simulink model "Planta_15_9_24"  (R2021a)
settings: Solver=VariableStepAuto  StartTime=0.0  StopTime=350  FixedStep=0.002  MaxStep=1e-3  RelTol=1e-4
model workspace (MAT data in the model file):
  VelMin = 0.5
  vMax = -0.3
values from neighbouring files (symbols this model uses):
  ax_max = 0.8    [valoresPlanta_29_9_24.m]    (also in valoresPlanta_v4.m)
  ay_max = 0.75    [valoresPlanta_29_9_24.m]    (also in valoresPlanta_v4.m)
  bcy = 1e7    (= 10000000)    [Valores_1.m]    (also in valoresPlanta.m; valoresPlanta_29_9_24.m; valoresPlanta_V3.m; valoresPlanta_v4.m)
  bh_eq = bhm*ih^2+bhd    (= 8720)    [Valores.m]    (also in Valores_1.m; valoresPlanta.m; valoresPlanta_29_9_24.m; valoresPlanta_V3.m)
  bhb = 1e8    (= 100000000)    [Valores.m]    (also in Valores_1.m; valoresPlanta.m; valoresPlanta_29_9_24.m; valoresPlanta_V3.m)
  bhEb = 2.2e9    (= 2200000000)    [Valores.m]    (also in Valores_1.m; valoresPlanta.m; valoresPlanta_29_9_24.m; valoresPlanta_V3.m)
  bt = 90.0    (= 90)    [Valores.m]    (also in Valores_1.m; valoresPlanta.m; valoresPlanta_29_9_24.m; valoresPlanta_V3.m)
  bt_eq = btd+(btm*(it^2))    (= 5401.8)    [valoresPlanta.m]    (also in valoresPlanta_29_9_24.m; valoresPlanta_V3.m; valoresPlanta_v4.m)
  btb = 5e6    (= 5000000)    [Valores.m]    (also in Valores_1.m; valoresPlanta.m; valoresPlanta_29_9_24.m; valoresPlanta_V3.m)
  btw = 3.0e3    (= 3000)    [Valores.m]    (also in Valores_1.m; valoresPlanta.m; valoresPlanta_29_9_24.m; valoresPlanta_V3.m)
  bwu = 150    [Valores.m]    (also in Valores_1.m; valoresPlanta.m; valoresPlanta_29_9_24.m; valoresPlanta_V3.m)
  estado_cont = [x_positions; hy_cont]    [perfilObsaculos.m]    (also in valoresPlanta_29_9_24.m = [x_positions; [hy_muelle hy_cont]]; valoresPlanta_v4.m = [x_positions; [hy_muelle hy_cont]])
  g = 9.80665    [Valores.m]    (also in Valores_1.m; valoresPlanta.m; valoresPlanta_29_9_24.m; valoresPlanta_V3.m)
  Hc = 0    [Valores.m]    (also in Valores_1.m = 2.5; valoresPlanta.m = 2.5; valoresPlanta_29_9_24.m = 2.5; valoresPlanta_V3.m = 2.5)
  hx_cont = 2.5    [perfilObsaculos.m]    (also in puntosTrayectoria.m; valoresPlanta_29_9_24.m; valoresPlanta_v4.m)
  ih = 22    [Valores.m]    (also in Valores_1.m; valoresPlanta.m; valoresPlanta_29_9_24.m; valoresPlanta_V3.m)
  it = 30    [Valores.m]    (also in Valores_1.m; valoresPlanta.m; valoresPlanta_29_9_24.m; valoresPlanta_V3.m)
  Jh_eq = Jhm_hb*ih^2+Jhd_hEb    (= 18320)    [Valores.m]    (also in Valores_1.m; valoresPlanta.m; valoresPlanta_29_9_24.m; valoresPlanta_V3.m)
  Jt_eq = Jtd+(Jtm_tb*(it^2))    (= 7500)    [valoresPlanta.m]    (also in valoresPlanta_29_9_24.m; valoresPlanta_V3.m; valoresPlanta_v4.m)
  kcy = 1.8e9    (= 1800000000)    [Valores_1.m]    (also in valoresPlanta.m; valoresPlanta_29_9_24.m; valoresPlanta_V3.m; valoresPlanta_v4.m)
  KDh = Jeq2 * w_posh^3    (= -12245.4404091)    [Valores.m]    (also in Valores_1.m = Jeq2 * w_posh; valoresPlanta.m = Jeq2 * w_posh; valoresPlanta_29_9_24.m = Jh_eq * n * w_posh; valoresPlanta_V3.m = Jeq2 * w_posh)
  KDt = Meq2 * w_post^3    (= -4728.86946035)    [Valores.m]    (also in Valores_1.m = Meq2 * w_post; valoresPlanta.m = Meq2 * w_post; valoresPlanta_29_9_24.m = 10127; valoresPlanta_V3.m = Meq2 * w_post)
  KIh = Jeq2 * w_posh^2    (= 2572.66592082)    [Valores.m]    (also in Valores_1.m = Jeq2 * w_posh^3; valoresPlanta.m = Jeq2 * w_posh^3; valoresPlanta_29_9_24.m = Jh_eq * w_posh^3; valoresPlanta_V3.m = Jeq2 * w_posh^3)
  KIt = Meq2 * w_post^2    (= 1307.690244)    [Valores.m]    (also in Valores_1.m = Meq2 * w_post^3; valoresPlanta.m = Meq2 * w_post^3; valoresPlanta_29_9_24.m = 6809.6; valoresPlanta_V3.m = Meq2 * w_post^3)
  KPh = Jeq2 * w_posh    (= -540.495867769)    [Valores.m]    (also in Valores_1.m = Jeq2 * w_posh^2; valoresPlanta.m = Jeq2 * w_posh^2; valoresPlanta_29_9_24.m = Jh_eq * n * w_posh^2; valoresPlanta_V3.m = Jeq2 * w_posh^2)
  KPt = Meq2 * w_post    (= -361.62)    [Valores.m]    (also in Valores_1.m = Meq2 * w_post^2; valoresPlanta.m = Meq2 * w_post^2; valoresPlanta_29_9_24.m = 14123; valoresPlanta_V3.m = Meq2 * w_post^2)
  Ktw = 4.8e5    (= 480000)    [Valores.m]    (also in Valores_1.m; valoresPlanta.m; valoresPlanta_29_9_24.m; valoresPlanta_V3.m)
  kwu = 2.36e8    (= 236000000)    [Valores.m]    (also in Valores_1.m; valoresPlanta.m; valoresPlanta_29_9_24.m; valoresPlanta_V3.m)
  Mc_max = 5e4    (= 50000)    [Valores.m]    (also in Valores_1.m; valoresPlanta.m; valoresPlanta_29_9_24.m; valoresPlanta_V3.m)
  Mc_min = 2e3    (= 2000)    [Valores.m]    (also in Valores_1.m; valoresPlanta.m; valoresPlanta_29_9_24.m; valoresPlanta_V3.m)
  Ms = 1.5e4    (= 15000)    [Valores.m]    (also in Valores_1.m; valoresPlanta.m; valoresPlanta_29_9_24.m; valoresPlanta_V3.m)
  Mt = 30000    [Valores.m]    (also in Valores_1.m; valoresPlanta.m; valoresPlanta_29_9_24.m; valoresPlanta_V3.m)
  pos = [p0; p1; p2; p3; p4; p5]    [calcularTrayectoria2_prueba.m]    (also in perfilObsaculos.m = puntosTrayectoria(4, 1.5, 20, [-20,0], estado_cont, hy_cont,; puntosTrayectoria.m; valoresPlanta_29_9_24.m = calcularTrayectoria2_prueba(vx_max, vhmax, ax_max, Hc, hx_co; valoresPlanta_v4.m = calcularTrayectoria2_prueba(vx_max, vhmax, ax_max, Hc, hx_co)
  rhd = 0.75    [Valores.m]    (also in Valores_1.m; valoresPlanta.m; valoresPlanta_29_9_24.m; valoresPlanta_V3.m)
  rtd = 0.5    [Valores.m]    (also in Valores_1.m; valoresPlanta.m; valoresPlanta_29_9_24.m; valoresPlanta_V3.m)
  tau_hm = 1e-3    (= 0.001)    [valoresPlanta.m]    (also in valoresPlanta_29_9_24.m; valoresPlanta_V3.m; valoresPlanta_v4.m)
  tau_tm = 1e-3    (= 0.001)    [Valores.m]    (also in Valores_1.m; valoresPlanta.m; valoresPlanta_29_9_24.m; valoresPlanta_V3.m)
  Thb_Max = 5e4    (= 50000)    [Valores.m]    (also in Valores_1.m; valoresPlanta.m; valoresPlanta_29_9_24.m; valoresPlanta_V3.m)
  ThEb_Max = 1.1e6    (= 1100000)    [Valores.m]    (also in Valores_1.m; valoresPlanta.m; valoresPlanta_29_9_24.m; valoresPlanta_V3.m)
  Thm_Max = 2e4    (= 20000)    [Valores.m]    (also in Valores_1.m; valoresPlanta.m; valoresPlanta_29_9_24.m; valoresPlanta_V3.m)
  Ttb_Max = 5e3    (= 5000)    [Valores.m]    (also in Valores_1.m; valoresPlanta.m; valoresPlanta_29_9_24.m; valoresPlanta_V3.m)
  Ttm_Max = 3e3    (= 3000)    [Valores.m]    (also in Valores_1.m; valoresPlanta.m; valoresPlanta_29_9_24.m = 4000; valoresPlanta_V3.m)
  vhmax = 3    [valoresPlanta_29_9_24.m]    (also in valoresPlanta_V3.m; valoresPlanta_v4.m)
  vx_max = 4    [valoresPlanta_29_9_24.m]    (also in valoresPlanta_v4.m)
  whmMax = P/Thm_Max    (= 47.8075)    [Valores_1.m]    (also in valoresPlanta.m; valoresPlanta_29_9_24.m = 176; valoresPlanta_V3.m; valoresPlanta_v4.m = 176)
  whmMin = 0.02    [valoresPlanta_29_9_24.m]    (also in valoresPlanta_v4.m = 0.2)
  wtmMax = (4/rtd)*it    (= 240)    [Valores_1.m]    (also in valoresPlanta.m; valoresPlanta_29_9_24.m; valoresPlanta_V3.m; valoresPlanta_v4.m)
  wtmMin = 0.02    [valoresPlanta_29_9_24.m]    (also in valoresPlanta_v4.m = 0.2)
  x_0 = -20    [valoresPlanta_29_9_24.m]    (also in valoresPlanta_v4.m)
  x_0_tamb = x_0/rtd    (= -40)    [valoresPlanta_29_9_24.m]    (also in valoresPlanta_v4.m)
  xLimMax = 49    [valoresPlanta_29_9_24.m]    (also in valoresPlanta_v4.m)
  xLimMaxSeguridad = 50    [valoresPlanta_29_9_24.m]    (also in valoresPlanta_v4.m)
  xLimMin = -29    [valoresPlanta_29_9_24.m]    (also in valoresPlanta_v4.m)
  xLimMinSeguridad = -30    [valoresPlanta_29_9_24.m]    (also in valoresPlanta_v4.m)
  y_0 = 2.5    [valoresPlanta_29_9_24.m]    (also in valoresPlanta_v4.m)
  y_0_izaje = 3*(2/rhd)    (= 8)    [valoresPlanta_29_9_24.m]    (also in valoresPlanta_v4.m)
  yLimMax = 44    [valoresPlanta_29_9_24.m]    (also in valoresPlanta_v4.m)
  yLimMaxSeguridad = 45    [valoresPlanta_29_9_24.m]    (also in valoresPlanta_v4.m)
  yLimMin = -19    [valoresPlanta_29_9_24.m]    (also in valoresPlanta_v4.m)
  yLimMinSeguridad = -20    [valoresPlanta_29_9_24.m]    (also in valoresPlanta_v4.m)
  Yt0 = 45    [Valores.m]    (also in Valores_1.m; valoresPlanta.m; valoresPlanta_29_9_24.m; valoresPlanta_V3.m)
undefined symbols (not defined in the file or in its folder): DiscIntNeverNeededParam
libraries: simulink x4, vrlib x1, simulink_extras x1, aerolibanimutils x1
(part 1 of 3)
settings Model: Creator=Matias  LastModifiedBy=agustin

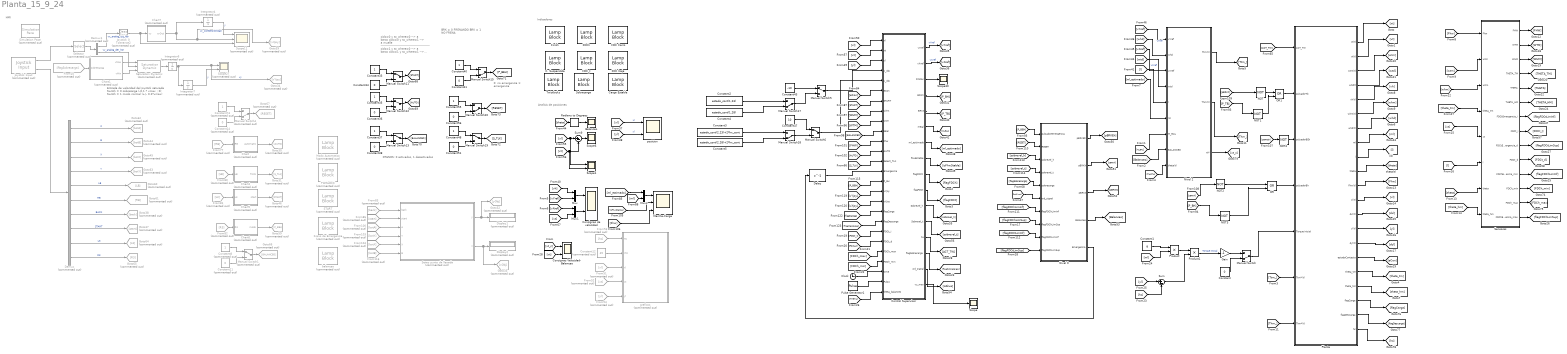
== system Planta_15_9_24 ==
  note: Entrada de velocidad del joystick saturada
      | Switch = 0 sobrecarga (-0.1 * vmax ; 0)
      | Switch = 1 modo normal (+/- 0.2*vmax)
  note: Indicadores
  note: Analisis de posiciones
  note: HMI
  note: 0: no emergencia
      | 1: emergencia
  note: ciclo=0 y to_where=0 --> a barco
      | ciclo=0 y to_where=1 --> a muelle
      | -------------------------------------------------
      | ciclo=1 y to_where=0 --> a barco
      | ciclo=1 y to_where=1 --> a barco 2
      | ciclo=1 y to_where=2 --> a muelle
  note: FRENOS: 0 activados, 1 desactivados
  note: BRK = 0 FRENANDO
      | BRK = 1 NO FRENA
  Balanceo : Scope
  C. Suspendida : LampBlock
  Carga Estable : LampBlock
  Chart : Stateflow chart  Commented=on  TreatAsAtomicUnit=on
  Chart1 : Stateflow chart  Commented=on  TreatAsAtomicUnit=on
  Chart4 : Stateflow chart  Commented=on  TreatAsAtomicUnit=on
  Chart5 : Stateflow chart  Commented=on  TreatAsAtomicUnit=on
  Chart6 : Stateflow chart  Commented=on  TreatAsAtomicUnit=on
  Chart7 : Stateflow chart  Commented=on  TreatAsAtomicUnit=on
  Clock : Clock
  Consignas Velocidad-Balanceo : Scope  NumInputPorts=2
  Consignas de velocidad : Scope  NumInputPorts=2
  Constant{,34,36,38,41,51,56} (7 alike) : Constant  Value=0
  Constant1 : Constant  Value=g
  Constant11 : Constant  Commented=on  Value=0
  Constant12 : Constant  Commented=on  Value=45
  Constant13 : Constant  Commented=on
  Constant14 : Constant  Commented=on  Value=0
  Constant2 : Constant  Value=estado_cont(1,23)
  Constant3 : Constant  Value=estado_cont(2,23)+2*hx_cont
  Constant{33,35,37,40,48,55} (6 alike) : Constant
  Constant4 : Constant  Value=estado_cont(1,28)
  Constant43 : Constant  Value=-10
  Constant47 : Constant  Value=10
  Constant5 : Constant  Value=estado_cont(2,28)+2*hx_cont
  Constant8 : Constant  Commented=on
  Control Supervisor : Subsystem  TreatAsAtomicUnit=on  SystemSampleTime=0.02
  Delay : Delay  DelayLength=1  InputProcessing=Columns as channels (frame based)
  Demux : Demux  Commented=on  Outputs=10
  Demux1 : Demux  Commented=on  Outputs=2
  Display1 : Display  Commented=on
  Display2 : Display  Commented=on
  FDC Carro : LampBlock
  FDC Izaje : LampBlock
  FDC_t : LampBlock
  FDCh : LampBlock
  Finish : LampBlock
  Freno de Emergencia : LampBlock  Commented=on  LabelPosition=Hide
  From10 : From  Commented=on  GotoTag=flagSobrecarga
  From100 : From  Commented=on  GotoTag=botA
  From103 : From  Commented=on  GotoTag=botY
  From104 : From  Commented=on  GotoTag=botX
  From116 : From  Commented=on  GotoTag=botB
  From51 : From  Commented=on  GotoTag=xl
  From52 : From  Commented=on  GotoTag=xt
  From53 : From  Commented=on  GotoTag=hc
  From54 : From  Commented=on  GotoTag=yl
  From77 : From  Commented=on  GotoTag=RB
  From80 : From  Commented=on  GotoTag=LB
  From81 : From  Commented=on  GotoTag=L3
  From82 : From  Commented=on  GotoTag=R3
  From83 : From  Commented=on  GotoTag=back
  From86 : From  Commented=on  GotoTag=start
  Gain : Gain  Gain=-1
  Goto30 : Goto  Commented=on  GotoTag=AUTO
  Goto31 : Goto  Commented=on  GotoTag=S_TLK
  Goto32 : Goto  Commented=on  GotoTag=yObj
  Goto33 : Goto  Commented=on  GotoTag=xObj
  Goto34 : Goto  Commented=on  GotoTag=vYjoy
  Goto37 : Goto  Commented=on  GotoTag=start
  Goto38 : Goto  Commented=on  GotoTag=back
  Goto39 : Goto  Commented=on  GotoTag=vXjoy
  Goto44 : Goto  Commented=on  GotoTag=botB
  Goto45 : Goto  Commented=on  GotoTag=botX
  Goto46 : Goto  Commented=on  GotoTag=START
  Goto59 : Goto  Commented=on  GotoTag=P_BEH
  Goto60 : Goto  Commented=on  GotoTag=LB
  Goto61 : Goto  Commented=on  GotoTag=RB
  Goto62 : Goto  Commented=on  GotoTag=botA
  Goto63 : Goto  Commented=on  GotoTag=botY
  Goto64 : Goto  Commented=on  GotoTag=L3
  Goto65 : Goto  Commented=on  GotoTag=R3
  Goto66 : Goto  Commented=on  GotoTag=BALANCEO
  Goto67 : Goto  Commented=on  GotoTag=RESET
  Integrator4 : Integrator  Commented=on
  Integrator6 : Integrator  Commented=on  InitialCondition=[0]  LimitOutput=on  UpperSaturationLimit=[3.5]  LowerSaturationLimit=[-3.5]
  Integrator7 : Integrator  Commented=on
  Joystick 0 Tolerance2 : DeadZone  Commented=on  LowerValue=-0.2  UpperValue=0.2  SaturateOnIntegerOverflow=on
  Joystick Input : vrlib/Joystick Input  Commented=on  joyid=1  adjustports=on  forcefeed=off
  Manual Switch{,15,17..18,20} (5 alike) : ManualSwitch  CurrentSetting=0
  Manual Switch1 : ManualSwitch  Commented=on
  Manual Switch{5..6,11..13,19} (6 alike) : ManualSwitch
  Manual Switch4 : ManualSwitch  Commented=on  CurrentSetting=0
  Marcha-Carga : Scope  NumInputPorts=3
  Modo Automatico : LampBlock  Commented=on  LabelPosition=Hide
  Mux : Mux  Inputs=2
  Mux1 : Mux  Inputs=2
  Mux2 : Mux  Inputs=2
  NOT{,1..4} (5 alike) : Logic  Operator=NOT  IconShape=distinctive  AllPortsSameDT=off  OutDataTypeStr=boolean
  Nivel 0 : Stateflow chart  TreatAsAtomicUnit=on  SystemSampleTime=0.02
  Nivel 2 : Subsystem  SystemSampleTime=0.005
  OR : Logic  Operator=OR  IconShape=distinctive  AllPortsSameDT=off  OutDataTypeStr=fixdt(0,1)
  OR1 : Logic  Operator=OR  IconShape=distinctive  AllPortsSameDT=off  OutDataTypeStr=fixdt(0,1)
  Planta : Subsystem
  Product : Product
  Product1 : Product
  Pulse Generator1 : DiscretePulseGenerator  PulseType=Time based  Period=1  PulseWidth=50
  Radians to Degrees : simulink_extras/Transformations/Radians to Degrees
  START : LampBlock  Commented=on  LabelPosition=Hide
  Saturation Dynamic : simulink/Discontinuities/Saturation Dynamic  Commented=on  OutMin=[]  OutMax=[]  OutDataTypeStr=Inherit: Same as second input  OutDataType=fixdt(1, 16)  OutScaling=2^-10  DoSatur=off
  Scope : Scope
  Scope1 : Scope  NumInputPorts=2
  Scope11 : Scope  Commented=on  NumInputPorts=3
  Scope27 : Scope  Commented=on  NumInputPorts=2
  Scope30 : Scope
  Scope6 : Scope
  Selector : Selector  Commented=on  InputPortWidth=5  IndexOptions=Index vector (dialog)  Indices=[1 4]  OutputSizes=1
  Sensores : Subsystem
  Seteo punto de llegada : Stateflow chart  Commented=on  TreatAsAtomicUnit=on
  Simulation Pace : aerolibanimutils/Simulation Pace  Commented=on  SimulationPace=1  SleepMode=Auto  OutputPaceError=off  SampleTime=1/50
  Sobrecarga : LampBlock
  Sum : Sum  Inputs=|+-
  Sum9 : Sum  Inputs=|+-
  TWISLOCK : LampBlock  Commented=on  LabelPosition=Hide
  Twistlocks : LampBlock
  balanceo : LampBlock  Commented=on  LabelPosition=Hide
  graficos : Stateflow chart  Commented=on  TreatAsAtomicUnit=on
  posicion : Scope  NumInputPorts=2
  wires:
  [xl] -> posicion/1  "xl"
  [yl] -> posicion/2  "yl"
  [yl] -> Control Supervisor/3(yl)
  Control Supervisor/2(vXref) -> [vXref]  "vXref"
  Control Supervisor/1(vYref) -> [vYref]  "vYref"
  [xl] -> Control Supervisor/1(xl)
  Constant12/1 -> graficos/2(Yt0)
  From52/1 -> graficos/4(xt)
  From51/1 -> graficos/3(xl)
  From53/1 -> graficos/1(Hc)
  From54/1 -> graficos/5(yl)
  [xl] -> Scope1/1, Sum9/1
  [xt] -> Sum9/2, Scope1/2
  Sum9/1 -> Scope6/1
  Radians to Degrees/1 -> Balanceo/1
  [theta] -> Radians to Degrees/1
  [xt] -> Control Supervisor/2(xt)
  [vh] -> Mux/1
  [vt] -> Mux1/2
  Mux1/1 -> Consignas de velocidad/2
  Mux/1 -> Consignas de velocidad/1
  [START] -> Control Supervisor/7(START)
  Control Supervisor/3(FINISH) -> Scope30/1
  [P_TB] -> NOT1/1
  [P_BH] -> NOT3/1
  [eCon] -> Control Supervisor/6(eCon)
  [WTM] -> Control Supervisor/9(wtm)
  [WHM] -> Control Supervisor/8(whm)
  [BALANCEO] -> Control Supervisor/10(bBal)
  Control Supervisor/6(mBal) -> [M_BAL]
  Control Supervisor/5(BRKt) -> [P_TB]
  Control Supervisor/4(BRKh) -> [P_BH]
  [FHW] -> Control Supervisor/11(Fhw)
  [AUTO] -> Control Supervisor/12(AUTO)
  [S_TLK] -> Control Supervisor/13(Select_TLK)
  Control Supervisor/7(ml_estimado) -> [ml_estimado]
  [ml] -> Mux2/2
  [ml_estimado] -> Mux2/1
  Control Supervisor/8(fhwEstable) -> [isFhwStable]
  [isFhwStable] -> Marcha-Carga/2
  [Fhw] -> Marcha-Carga/3
  [P_BEH] -> Nivel 0/1(pulsadorEmergencia)
  Nivel 0/3(pBRKt) -> [pBRKt]
  Nivel 0/2(pBRKh) -> [pBRKh]
  Nivel 0/1(pBRKEh) -> [pBRKEh]
  [pBRKh] -> NOT2/1
  [pBRKt] -> NOT/1
  Nivel 0/4(Balanceo) -> [Balanceo]
  Control Supervisor/9(flagFDCh) -> [flagFDCh]
  Control Supervisor/10(flagFDCt) -> [flagFDCt]
  [RESET] -> Nivel 0/2(RESET)
  Control Supervisor/11(Sobrevel_h) -> [sobrevel_h]
  Control Supervisor/12(Sobrevel_t) -> [sobrevel_t]
  [sobrevel_t] -> Nivel 0/4(sobrevel_t)
  [sobrevel_h] -> Nivel 0/3(sobrevel_h)
  Delay/1 -> Control Supervisor/14(Emergencia)
  [P_BEH] -> Control Supervisor/15(P_EH)
  Nivel 0/5(Emergencia) -> Delay/1
  Control Supervisor/13(tw) -> [ACT_TW]
  [flagSobrecarga] -> Nivel 0/5(sobrecarga)
  From83/1 -> Seteo punto de llegada/1(back)
  From86/1 -> Seteo punto de llegada/2(start)
  Chart7/1(vyOut) -> Goto39/1, Scope11/2, Integrator4/1  "vy_conSensibilidad"
  Seteo punto de llegada/1(y) -> Goto32/1, Display1/1
  Seteo punto de llegada/2(x) -> Goto33/1, Display2/1
  Chart4/1(TWIS) -> Goto31/1
  From100/1 -> Seteo punto de llegada/3(A)
  From104/1 -> Seteo punto de llegada/5(X)
  Demux/9 -> Goto64/1  "L3"
  From103/1 -> Seteo punto de llegada/4(Y)
  Selector/1 -> Demux1/1
  Integrator7/1 -> Scope27/2  "y"
  Integrator4/1 -> Scope11/1  "y"
  Demux1/2 -> Saturation Dynamic/2  "vy_analog_der_hor"
  From80/1 -> Chart4/1(LB)
  Demux1/1 -> Joystick 0 Tolerance2/1  "vx_analog_izq_hor"
  Demux/5 -> Goto60/1  "LB"
  From81/1 -> Chart5/1(L3)
  From82/1 -> Chart6/1(R3)
  Chart5/1(start) -> Goto46/1
  Saturation Dynamic/1 -> Integrator6/1
  Integrator6/1 -> Integrator7/1, Goto34/1, Scope27/1  "vy"
  Demux/10 -> Goto65/1  "R3"
  Chart/1(automatic) -> Goto30/1
  Joystick Input/1 -> Selector/1
  Chart6/1(modo) -> Goto59/1
  From77/1 -> Chart/1(RB)
  Demux/8 -> Goto37/1  "START"
  Demux/3 -> Goto45/1  "X"
  From116/1 -> Seteo punto de llegada/6(B)
  Demux/4 -> Goto63/1  "Y"
  Joystick Input/2 -> Demux/1
  Demux/6 -> Goto61/1  "RB"
  Demux/7 -> Goto38/1  "BACK"
  Demux/1 -> Goto62/1  "A"
  Demux/2 -> Goto44/1  "B"
  Joystick 0 Tolerance2/1 -> Scope11/3, Chart7/1(vy)
  Manual Switch1/1 -> Goto66/1
  Constant8/1 -> Manual Switch1/1
  Constant11/1 -> Manual Switch1/2
  Manual Switch4/1 -> Goto67/1
  Constant14/1 -> Manual Switch4/2
  Constant13/1 -> Manual Switch4/1
  [vYjoy] -> Control Supervisor/16(vYjoy)
  [vXjoy] -> Control Supervisor/17(vXjoy)
  [flagCarga] -> Control Supervisor/18(flagCarga)
  Control Supervisor/14(flagSobrecarga) -> [flagSobrecarga]
  Control Supervisor/15(wd_signal) -> [isAlive]
  [isAlive] -> Nivel 0/6(wd_signal)
  Manual Switch11/1 -> [START]
  Constant56/1 -> Manual Switch20/2
  Constant51/1 -> Manual Switch19/2
  Manual Switch19/1 -> [S_TLK]
  Constant37/1 -> Manual Switch13/1
  Constant48/1 -> Manual Switch19/1
  Constant55/1 -> Manual Switch20/1
  Manual Switch12/1 -> [AUTO]
  Manual Switch13/1 -> [BALANCEO]
  Constant40/1 -> Manual Switch15/1
  Manual Switch20/1 -> [RESET]
  Constant41/1 -> Manual Switch15/2
  Constant36/1 -> Manual Switch12/2
  Constant33/1 -> Manual Switch11/1
  Manual Switch15/1 -> [P_BEH]
  Constant35/1 -> Manual Switch12/1
  Constant34/1 -> Manual Switch11/2
  Constant38/1 -> Manual Switch13/2
  Constant2/1 -> Manual Switch17/1
  Constant3/1 -> Manual Switch18/1
  Constant43/1 -> Manual Switch5/1
  Manual Switch17/1 -> Manual Switch5/2
  Manual Switch5/1 -> Control Supervisor/4(x_obj)
  Manual Switch6/1 -> Control Supervisor/5(y_obj)
  Manual Switch18/1 -> Manual Switch6/2
  Constant47/1 -> Manual Switch6/1
  [flagDescarga] -> Control Supervisor/19(flagDescarga)
  [ACT_TW] -> Planta/1(ACT_TW)
  Planta/1(xt(t)) -> [xt]
  Planta/2(vt(t)) -> [vt]
  Planta/3(wtm(t)) -> [wtm]
  Planta/4(wtd(t)) -> [wtd]
  Planta/5(vh(t)) -> [vh]
  Planta/6(whm(t)) -> [whm]
  Planta/7(whd(t)) -> [whd]
  Planta/8(ml) -> [ml]
  Planta/9(l) -> [l]
  Planta/10(theta) -> [theta]
  Planta/11(Fhw(t)) -> [Fhw]
  Planta/12(xl(t)) -> [xl]
  Planta/13(dxl(t)) -> [dxl]
  Planta/14(yl(t)) -> [yl]
  Planta/15(dyl(t)) -> [dyl]
  [pBRKEh] -> NOT4/1
  OR/1 -> Planta/4(pulsadorBh)
  OR1/1 -> Planta/2(pulsadorTb)
  [vYref] -> Nivel 2/1(vYref)  "vYref"
  [whd] -> Nivel 2/2(whd)
  [vXref] -> Nivel 2/3(vXref)  "vXref"
  [wtd] -> Nivel 2/4(wtd)
  [ml_estimado] -> Nivel 2/6(ml)
  Nivel 2/1(Ttm(t)) -> [Ttm_]
  Nivel 2/2(Thm(t)) -> [Thm_]
  [l] -> Nivel 2/5(l)
  [Balanceo] -> Nivel 2/8(BALANCEO)
  [M_BAL] -> Nivel 2/7(M_BAL)
  [vYref] -> Mux/2
  [vXref] -> Mux1/1
  Planta/16(estadoContacto) -> [eCon]
  [Fhw] -> Sensores/1(Fhw)
  From10/1 -> Chart1/1(sobreCarga)
  Chart1/1(vMax) -> Saturation Dynamic/1
  Chart1/2(vMin) -> Saturation Dynamic/3
  [wtm] -> Sensores/2(wtm)
  [whm] -> Sensores/3(whm)
  [theta] -> Sensores/7(theta)
  Planta/18(theta_hm) -> [theta_hm]
  Planta/17(theta_tm) -> [theta_tm]
  [theta_tm] -> Sensores/4(theta_tm)
  [theta_hm] -> Sensores/8(theta_hm)
  [xt] -> Sensores/5(xt)
  [l] -> Sensores/6(l)
  Sensores/1(FHW) -> [FHW]
  Sensores/2(WTM) -> [WTM]
  Sensores/3(WHM) -> [WHM]
  Sensores/4(THETA_TM) -> [THETA_TM]
  Sensores/5(THETA) -> [THETA]
  Sensores/6(THETA_HM) -> [THETA_HM]
  [flagFDChLimInf] -> Nivel 0/7(flagFDChLimInf)
  [flagFDChLimSup] -> Nivel 0/8(flagFDChLimSup)
  [flagFDCtLimInf] -> Nivel 0/9(flagFDCtLimInf)
  [flagFDCtLimSup] -> Nivel 0/10(flagFDCtLimSup)
  Sensores/11(FDChEmergencia_min) -> [flagFDChLimInf]
  Sensores/9(FDCtEmergencia_d) -> [flagFDCtLimSup]
  Sensores/7(FDCtEmergencia_i) -> [flagFDCtLimInf]
  Sensores/14(FDChEmergencia_max) -> [flagFDChLimSup]
  Sensores/13(FDCh_max) -> [FDCh_max]
  Sensores/12(FDCh_min) -> [FDCh_min]
  Sensores/10(FDCt_d) -> [FDCt_d]
  Sensores/8(FDCt_i) -> [FDCt_i]
  [FDCt_i] -> Control Supervisor/20(FDCt_i)
  [FDCt_d] -> Control Supervisor/21(FDCt_d)
  [FDCh_max] -> Control Supervisor/22(FDCh_max)
  [FDCh_min] -> Control Supervisor/23(FDCh_min)
  Planta/19(flagCarga) -> [flagCarga]
  Planta/20(flagDescarga) -> [flagDescarga]
  Constant1/1 -> Product/1
  [ml] -> Product/2
  Product/1 -> Product1/1
  [yl] -> Sum/1
  [hc] -> Sum/2
  Sum/1 -> Product1/2
  Product1/1 -> Gain/1  "Torque Inicial"
  Planta/21(hc) -> [hc]
  Manual Switch/1 -> Planta/5(Torque Inicial)
  Constant/1 -> Manual Switch/2
  Gain/1 -> Manual Switch/1
  NOT1/1 -> OR1/2
  NOT/1 -> OR1/1
  NOT3/1 -> OR/2
  NOT2/1 -> OR/1
  NOT4/1 -> Planta/3(pulsadorBEh)
  Clock/1 -> Control Supervisor/24(time)
  Pulse Generator1/1 -> Control Supervisor/25(Pulso)
  [Thm_] -> Planta/7(Thm*(t))
  [Ttm_] -> Planta/6(Ttm*(t))
  Control Supervisor/16(vy_max) -> Scope/1
  [THETA] -> Nivel 2/9(theta(t))
  [THETA] -> Control Supervisor/26(theta_balanceo)
  Nivel 2/3(xt*) -> [xt_c]
  [xt_c] -> Consignas Velocidad-Balanceo/1
  [vt] -> Consignas Velocidad-Balanceo/2
  Mux2/1 -> Marcha-Carga/1
  Constant5/1 -> Manual Switch18/2
  Constant4/1 -> Manual Switch17/2

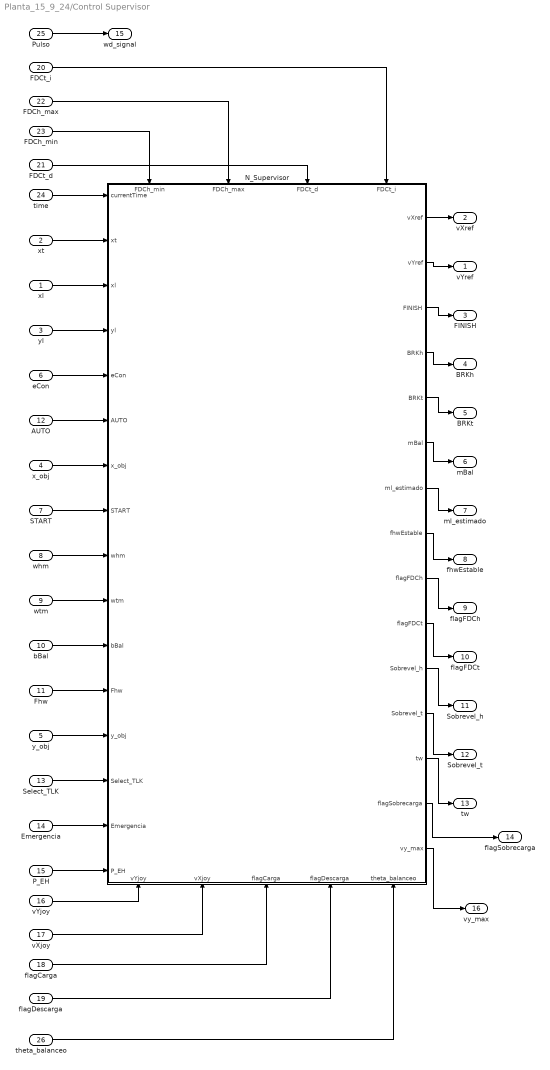
== system Planta_15_9_24/Control Supervisor ==
  xl : Inport
  xt : Inport  Port=2
  yl : Inport  Port=3
  x_obj : Inport  Port=4
  y_obj : Inport  Port=5
  eCon : Inport  Port=6
  START : Inport  Port=7
  whm : Inport  Port=8
  wtm : Inport  Port=9
  bBal : Inport  Port=10
  Fhw : Inport  Port=11
  AUTO : Inport  Port=12
  Select_TLK : Inport  Port=13
  Emergencia : Inport  Port=14
  P_EH : Inport  Port=15
  vYjoy : Inport  Port=16
  vXjoy : Inport  Port=17
  flagCarga : Inport  Port=18
  flagDescarga : Inport  Port=19
  FDCt_i : Inport  Port=20
  FDCt_d : Inport  Port=21
  FDCh_max : Inport  Port=22
  FDCh_min : Inport  Port=23
  time : Inport  Port=24
  Pulso : Inport  Port=25
  theta_balanceo : Inport  Port=26
  N_Supervisor : Stateflow chart  TreatAsAtomicUnit=on
      settings: PortSchema="{\"entries\":[{\"content\":{\"sides\":[{\"content\":{\"connectorIds\":[\"In13\",\"In11\",\"In8\",\"In10\",\"In12\",\"In19\",\"In20\",\"In14\",\"In15\",\"In16\",\"In17\",\"In18\",\"In21\",\"In22\",\"In23\",\"In24\"]},\"type\":\"ConnectorPlacement.EquallySpacedRectSide\",\"uuid\":\"7754e6e1-1487-4c5e-b93c-5b95548dc503\"},{\"content\":{\"connectorIds\":[\"Out1\",\"Out2\",\"Out3\",\"Out4\",\"Out5\",\"Out6\",\"Out7\",\"Out8\",\"Out9\",\"Out10\",\"Out11\",\"Out12\",\"Out13\",\"Out14\",\"Out15\"],\"side\":\"RIGHT\"},\"type\":\"ConnectorPlacement.EquallySpacedRectSide\",\"uuid\":\"e49bdf6e-b30d-4ce2-b56a-406d79434d70\"},{\"content\":{\"connectorIds\":[\"In1\",\"In2\",\"In3\",\"In4\"],\"side\":\"TOP\"},\"type\":\"ConnectorPlacement.EquallySpacedRectSide\",\"uuid\":\"816dde99-88b4-4e51-8e7c-8334ef27840c\"},{\"content\":{\"connectorIds\":[\"In6\",\"In7\",\"In25\",\"In9\",\"In5\"],\"side\":\"BOTTOM\"},\"type\":\"ConnectorPlacement.EquallySpacedRectSide\",\"uuid\":\"e82c3757-072b-4fbd-890b-1ff74979e1d6\"}]},\"type\":\"ConnectorPlacement.EquallySpacedConnector\",\"uuid\":\"e43ca6b0-ace3-4be2-8389-da1b8832a6a4\"}],\"packageUris\":[\"http://schema.mathworks.com/mf0/Connector/R2020b\"],\"version\":\"1.0\"}"
  vYref : Outport
  vXref : Outport  Port=2
  FINISH : Outport  Port=3
  BRKh : Outport  Port=4
  BRKt : Outport  Port=5
  mBal : Outport  Port=6
  ml_estimado : Outport  Port=7
  fhwEstable : Outport  Port=8
  flagFDCh : Outport  Port=9
  flagFDCt : Outport  Port=10
  Sobrevel_h : Outport  Port=11
  Sobrevel_t : Outport  Port=12
  tw : Outport  Port=13
  flagSobrecarga : Outport  Port=14
  wd_signal : Outport  Port=15
  vy_max : Outport  Port=16
  wires:
  N_Supervisor/3(FINISH) -> FINISH/1
  flagCarga/1 -> N_Supervisor/25(flagCarga)
  N_Supervisor/8(fhwEstable) -> fhwEstable/1
  flagDescarga/1 -> N_Supervisor/9(flagDescarga)
  N_Supervisor/4(BRKh) -> BRKh/1
  N_Supervisor/9(flagFDCh) -> flagFDCh/1
  Pulso/1 -> wd_signal/1
  FDCh_max/1 -> N_Supervisor/2(FDCh_max)
  N_Supervisor/6(mBal) -> mBal/1
  N_Supervisor/13(tw) -> tw/1
  FDCt_i/1 -> N_Supervisor/4(FDCt_i)
  time/1 -> N_Supervisor/13(currentTime)
  N_Supervisor/2(vYref) -> vYref/1
  FDCh_min/1 -> N_Supervisor/1(FDCh_min)
  N_Supervisor/1(vXref) -> vXref/1
  Emergencia/1 -> N_Supervisor/23(Emergencia)
  FDCt_d/1 -> N_Supervisor/3(FDCt_d)
  Fhw/1 -> N_Supervisor/18(Fhw)
  P_EH/1 -> N_Supervisor/24(P_EH)
  vXjoy/1 -> N_Supervisor/7(vXjoy)
  vYjoy/1 -> N_Supervisor/6(vYjoy)
  whm/1 -> N_Supervisor/15(whm)
  N_Supervisor/14(flagSobrecarga) -> flagSobrecarga/1
  N_Supervisor/5(BRKt) -> BRKt/1
  N_Supervisor/12(Sobrevel_t) -> Sobrevel_t/1
  eCon/1 -> N_Supervisor/12(eCon)
  N_Supervisor/11(Sobrevel_h) -> Sobrevel_h/1
  xt/1 -> N_Supervisor/11(xt)
  bBal/1 -> N_Supervisor/17(bBal)
  xl/1 -> N_Supervisor/8(xl)
  N_Supervisor/10(flagFDCt) -> flagFDCt/1
  wtm/1 -> N_Supervisor/16(wtm)
  N_Supervisor/7(ml_estimado) -> ml_estimado/1
  AUTO/1 -> N_Supervisor/19(AUTO)
  Select_TLK/1 -> N_Supervisor/22(Select_TLK)
  x_obj/1 -> N_Supervisor/20(x_obj)
  yl/1 -> N_Supervisor/10(yl)
  y_obj/1 -> N_Supervisor/21(y_obj)
  START/1 -> N_Supervisor/14(START)
  N_Supervisor/15(vy_max) -> vy_max/1
  theta_balanceo/1 -> N_Supervisor/5(theta_balanceo)

== system Planta_15_9_24/Nivel 2 ==
  vYref : Inport
  whd : Inport  Port=2
  vXref : Inport  Port=3
  wtd : Inport  Port=4
  l : Inport  Port=5
  ml : Inport  Port=6
  M_BAL : Inport  Port=7
  BALANCEO : Inport  Port=8
  theta(t) : Inport  Port=9
  Subsystem1 : Subsystem  TreatAsAtomicUnit=on  SystemSampleTime=0.005
  Ttm(t) : Outport
  Thm(t) : Outport  Port=2
  xt* : Outport  Port=3
  wires:
  vYref/1 -> Subsystem1/1(vYref)
  M_BAL/1 -> Subsystem1/7(M_BAL)
  whd/1 -> Subsystem1/2(whd)
  BALANCEO/1 -> Subsystem1/8(BALANCEO)
  vXref/1 -> Subsystem1/3(vXref)
  wtd/1 -> Subsystem1/4(wtd)
  l/1 -> Subsystem1/5(l)
  ml/1 -> Subsystem1/6(ml)
  Subsystem1/2(Thm_) -> Thm(t)/1
  Subsystem1/1(Ttm_) -> Ttm(t)/1
  theta(t)/1 -> Subsystem1/9(theta(t))
  Subsystem1/3(xt*) -> xt*/1

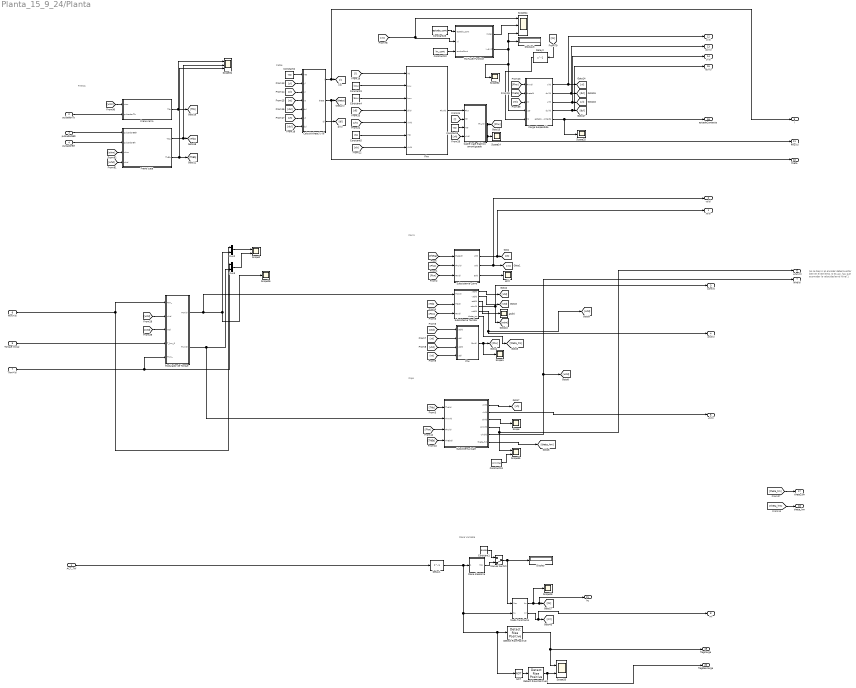
== system Planta_15_9_24/Planta ==
  note: No se bien si el encoder debería estar bien en el eje lento. Si es asi, hay que acomodar la velocidad en el Nivel 1
  note: Masa Variable
  note: Cable
  note: Izaje
  note: Carro
  note: Frenos
  ACT_TW : Inport
  pulsadorTb : Inport  Port=2
  pulsadorBEh : Inport  Port=3
  pulsadorBh : Inport  Port=4
  Torque Inicial : Inport  Port=5
  Ttm*(t) : Inport  Port=6
  Thm*(t) : Inport  Port=7
  Cable izaje elástico amortiguado : Subsystem
  Calculo theta,l y dl : Subsystem
  Carga Suspendida : Subsystem
  Constant1 : Constant  Value=50000
  Constant19 : Constant  Value=whmMax
  Constant2 : Constant  Value=Yt0
  Constant22 : Constant  Value=hx_cont
  Constant23 : Constant  Value=estado_cont
  Constant3 : Constant  Value=kwu
  Constant4 : Constant  Value=bwu
  Constant5 : Constant  Value=Yt0
  Constant6 : Constant  Value=Yt0
  Delay1 : Delay  DelayLength=1  InputProcessing=Columns as channels (frame based)
  Delay2 : Delay  DelayLength=1  InputProcessing=Columns as channels (frame based)
  Detect Rise Positive : simulink/Logic and Bit Operations/Detect Rise Positive  vinit=0  OutDataTypeStr=boolean
  Detect Rise Positive1 : simulink/Logic and Bit Operations/Detect Rise Positive  vinit=0  OutDataTypeStr=boolean
  Display : Display
  Display3 : Display
  Fhw : Subsystem
  Freno Izaje : Subsystem
  Freno carro : Subsystem
  Ftw : Subsystem
  MATLAB Function : MATLAB Function  TreatAsAtomicUnit=on
  Manual Switch : ManualSwitch  CurrentSetting=0
  Masa Aleatoria : Stateflow chart  TreatAsAtomicUnit=on
  Modo Twistlocks : Stateflow chart  TreatAsAtomicUnit=on
  Modulador de Torque : Subsystem
  Mux2 : Mux  Inputs=2
  Mux3 : Mux  Inputs=2
  NOT : Logic  Operator=NOT  IconShape=distinctive  AllPortsSameDT=off  OutDataTypeStr=boolean
  Scope{,1,14,25..26,28,32} (7 alike) : Scope
  Scope2 : Scope  NumInputPorts=2
  Scope24 : Scope  NumInputPorts=3
  Scope31 : Scope  NumInputPorts=3
  Scope33 : Scope  NumInputPorts=2
  Scope35 : Scope  NumInputPorts=2
  Subsistema Carro : Subsystem
  Subsistema Izaje : Subsystem
  Subsistema Tambor : Subsystem
  at(t) : Scope
  atd(t) : Scope
  xt(t) : Outport
  vt(t) : Outport  Port=2
  wtm(t) : Outport  Port=3
  wtd(t) : Outport  Port=4
  vh(t) : Outport  Port=5
  whm(t) : Outport  Port=6
  whd(t) : Outport  Port=7
  ml : Outport  Port=8
  l : Outport  Port=9
  theta : Outport  Port=10
  Fhw(t) : Outport  Port=11
  xl(t) : Outport  Port=12
  dxl(t) : Outport  Port=13
  yl(t) : Outport  Port=14
  dyl(t) : Outport  Port=15
  estadoContacto : Outport  Port=16
  theta_tm : Outport  Port=17
  theta_hm : Outport  Port=18
  flagCarga : Outport  Port=19
  flagDescarga : Outport  Port=20
  hc : Outport  Port=21
  wires:
  Fhw/1(Fhw(t)) -> Cable izaje elástico amortiguado/1(Fhw)
  Modo Twistlocks/1(hc) -> Scope28/1, hc/1, [hc]
  Subsistema Tambor/2(vtd(t)) -> [vtd]
  Constant23/1 -> MATLAB Function/1(estado_cont)
  [l] -> Fhw/1(l(t))
  [theta] -> Carga Suspendida/2(theta(t))
  [vh] -> Fhw/5(vh(t))
  [hc] -> Delay2/1
  Subsistema Carro/1(xt(t)) -> xt(t)/1, [xt]
  [ml] -> Carga Suspendida/3(ml)
  [dl] -> Fhw/4(dl(t))
  Subsistema Izaje/5(whd(t)) -> [whd], whd(t)/1
  Cable izaje elástico amortiguado/1(Fhw(t)) -> Scope14/1, Fhw(t)/1, [Fhw]
  Carga Suspendida/4(dyl(t)) -> dyl(t)/1, [dyl]
  Constant5/1 -> Fhw/6(Yt0)
  Subsistema Izaje/3(ah(t)) -> Scope/1
  [xt] -> Scope24/1, MATLAB Function/2(xl)
  Subsistema Izaje/2(vh(t)) -> vh(t)/1
  Subsistema Izaje/4(whm(t)) -> Scope35/1, whm(t)/1
  Carga Suspendida/2(dxl(t)) -> dxl(t)/1, [dxl]
  Carga Suspendida/5(estadoContacto) -> Scope25/1, estadoContacto/1
  Ftw/1(Ftw(t)) -> Scope1/1, [Ftw]
  [Fhw] -> Carga Suspendida/1(Fhw(t))
  Subsistema Izaje/1(xh(t)) -> [xh]
  [xt] -> Ftw/2(xt(t))
  Delay2/1 -> Carga Suspendida/5(hc)
  Delay1/1 -> Modo Twistlocks/2(tw), NOT/1, Detect Rise Positive/1, Masa Aleatoria/1(modo_tw)
  [theta] -> Subsistema Carro/1(theta(t))
  [dyl] -> Calculo theta,l y dl/7(dyl)
  [xtd] -> Ftw/1(xtd(t))
  Subsistema Carro/3(at(t)) -> at(t)/1
  [dxl] -> Calculo theta,l y dl/5(dxl)
  Subsistema Carro/2(vt(t)) -> vt(t)/1, [vt]
  [Ftw] -> Subsistema Carro/3(Ftw(t))
  [vtd] -> Ftw/3(vtd(t))
  [vt] -> Ftw/4(vt(t))
  Subsistema Tambor/3(atd(t)) -> atd(t)/1
  [Fhw] -> Subsistema Izaje/3(Fhw(t))
  [xh] -> Cable izaje elástico amortiguado/4(xh(t))
  Constant4/1 -> Fhw/3(bwu)
  Manual Switch/1 -> Display/1, Modo Twistlocks/1(Mcx)
  Calculo theta,l y dl/1(l) -> l/1, [l]
  [vt] -> Calculo theta,l y dl/6(vt)
  [yl] -> Calculo theta,l y dl/2(yl)
  Carga Suspendida/1(xl(t)) -> xl(t)/1, [xl]
  Constant6/1 -> Cable izaje elástico amortiguado/3(Yt0)
  Detect Rise Positive1/1 -> flagDescarga/1, Scope33/2
  Calculo theta,l y dl/3(dl) -> [dl]
  Subsistema Tambor/1(xtd(t)) -> [xtd]
  Constant2/1 -> Calculo theta,l y dl/1(Yt0)
  [xt] -> Calculo theta,l y dl/4(xt)
  MATLAB Function/1(index) -> Scope24/2
  Calculo theta,l y dl/2(theta) -> theta/1, [theta]
  Constant3/1 -> Fhw/2(kwu)
  Carga Suspendida/3(yl(t)) -> yl(t)/1, [yl]
  [xl] -> Calculo theta,l y dl/3(xl)
  [l] -> Cable izaje elástico amortiguado/2(l(t))
  [Ftw] -> Subsistema Tambor/3(Ftw(t))
  [Fhw] -> Subsistema Carro/2(Fhw(t))
  Constant1/1 -> Manual Switch/1
  Constant22/1 -> MATLAB Function/3(anchoCont)
  [Ttb] -> Subsistema Tambor/2(Ttb(t))
  MATLAB Function/2(y_evol) -> Carga Suspendida/4(yc0), Scope32/1, Display3/1, Scope24/3
  Masa Aleatoria/1(Mcx) -> Manual Switch/2
  Modo Twistlocks/2(ml) -> ml/1, [ml]
  [xh] -> Fhw/7(xh(t))
  Subsistema Tambor/5(wtd(t)) -> [wtd], wtd(t)/1
  Subsistema Tambor/4(wtm(t)) -> [wtm], wtm(t)/1
  Detect Rise Positive/1 -> flagCarga/1, Scope33/1
  NOT/1 -> Detect Rise Positive1/1
  Constant19/1 -> Scope35/2
  ACT_TW/1 -> Delay1/1
  Freno Izaje/1(Thb) -> Scope31/2, [Thb]
  [whd] -> Freno Izaje/4(whd)
  pulsadorBh/1 -> Freno Izaje/2(pulsadorBh)
  Freno carro/1(Ttb) -> Scope31/1, [Ttb]
  pulsadorBEh/1 -> Freno Izaje/1(pulsadorBEh)
  [whm] -> Freno Izaje/3(whm)
  Freno Izaje/2(ThEb) -> Scope31/3, [ThEb]
  [wtm] -> Freno carro/1(wtm)
  [Thb] -> Subsistema Izaje/1(Thb(t))
  [ThEb] -> Subsistema Izaje/4(ThEb(t))
  pulsadorTb/1 -> Freno carro/2(pulsadorTb)
  Subsistema Tambor/6(theta_tm) -> [theta_tm]
  Subsistema Izaje/6(theta_hm) -> [theta_hm]
  [theta_hm] -> theta_hm/1
  [theta_tm] -> theta_tm/1
  Mux2/1 -> Scope2/1
  Thm*(t)/1 -> Modulador de Torque/5(Thm_), Mux3/1
  Mux3/1 -> Scope2/2
  Ttm*(t)/1 -> Modulador de Torque/1(Ttm_), Mux2/1
  Modulador de Torque/2(Thm(t)) -> Subsistema Izaje/2(Thm(t)), Mux3/2
  Modulador de Torque/1(Ttm(t)) -> Subsistema Tambor/1(Ttm(t)), Scope26/1, Mux2/2
  Torque Inicial/1 -> Modulador de Torque/4(T_hm_0)
  [whd] -> Modulador de Torque/2(whd)
  [wtd] -> Modulador de Torque/3(wtd)

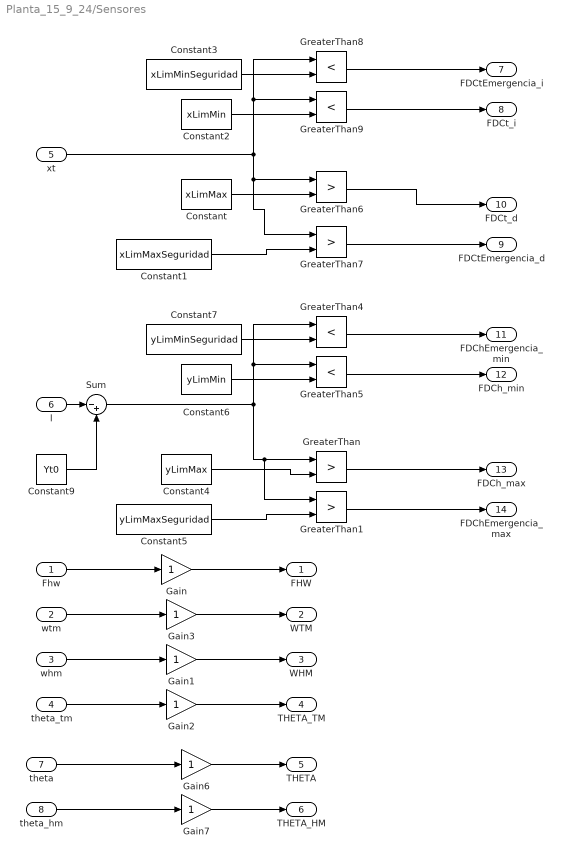
== system Planta_15_9_24/Sensores ==
  Fhw : Inport
  wtm : Inport  Port=2
  whm : Inport  Port=3
  theta_tm : Inport  Port=4
  xt : Inport  Port=5
  l : Inport  Port=6
  theta : Inport  Port=7
  theta_hm : Inport  Port=8
  Constant : Constant  Value=xLimMax
  Constant1 : Constant  Value=xLimMaxSeguridad
  Constant2 : Constant  Value=xLimMin
  Constant3 : Constant  Value=xLimMinSeguridad
  Constant4 : Constant  Value=yLimMax
  Constant5 : Constant  Value=yLimMaxSeguridad
  Constant6 : Constant  Value=yLimMin
  Constant7 : Constant  Value=yLimMinSeguridad
  Constant9 : Constant  Value=Yt0
  Gain{,1..3,6..7} (6 alike) : Gain
  GreaterThan{,1,6..7} (4 alike) : RelationalOperator  Operator=>  OutDataTypeStr=boolean  RndMeth=Simplest
  GreaterThan{4..5,8..9} (4 alike) : RelationalOperator  Operator=<  OutDataTypeStr=boolean  RndMeth=Simplest
  Sum : Sum  Inputs=|-+
  FHW : Outport
  WTM : Outport  Port=2
  WHM : Outport  Port=3
  THETA_TM : Outport  Port=4
  THETA : Outport  Port=5
  THETA_HM : Outport  Port=6
  FDCtEmergencia_i : Outport  Port=7
  FDCt_i : Outport  Port=8
  FDCtEmergencia_d : Outport  Port=9
  FDCt_d : Outport  Port=10
  FDChEmergencia_min : Outport  Port=11
  FDCh_min : Outport  Port=12
  FDCh_max : Outport  Port=13
  FDChEmergencia_max : Outport  Port=14
  wires:
  Fhw/1 -> Gain/1
  Gain/1 -> FHW/1
  theta_hm/1 -> Gain7/1
  theta/1 -> Gain6/1
  theta_tm/1 -> Gain2/1
  whm/1 -> Gain1/1
  wtm/1 -> Gain3/1
  Gain3/1 -> WTM/1
  Gain1/1 -> WHM/1
  Gain2/1 -> THETA_TM/1
  Gain6/1 -> THETA/1
  Gain7/1 -> THETA_HM/1
  Sum/1 -> GreaterThan1/1, GreaterThan/1, GreaterThan4/1, GreaterThan5/1
  Constant5/1 -> GreaterThan1/2
  Constant4/1 -> GreaterThan/2
  Constant6/1 -> GreaterThan5/2
  Constant1/1 -> GreaterThan7/2
  Constant2/1 -> GreaterThan9/2
  xt/1 -> GreaterThan8/1, GreaterThan9/1, GreaterThan6/1, GreaterThan7/1
  GreaterThan8/1 -> FDCtEmergencia_i/1
  GreaterThan9/1 -> FDCt_i/1
  GreaterThan6/1 -> FDCt_d/1
  GreaterThan7/1 -> FDCtEmergencia_d/1
  GreaterThan4/1 -> FDChEmergencia_min/1
  GreaterThan5/1 -> FDCh_min/1
  GreaterThan/1 -> FDCh_max/1
  GreaterThan1/1 -> FDChEmergencia_max/1
  l/1 -> Sum/1
  Constant9/1 -> Sum/2
  Constant7/1 -> GreaterThan4/2
  Constant/1 -> GreaterThan6/2
  Constant3/1 -> GreaterThan8/2

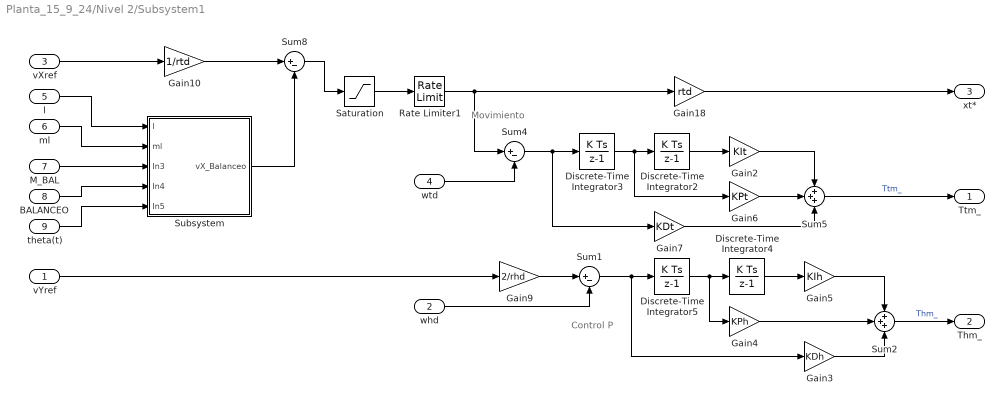
== system Planta_15_9_24/Nivel 2/Subsystem1 ==
  note: Movimiento
  note: Control P
  vYref : Inport
  whd : Inport  Port=2
  vXref : Inport  Port=3
  wtd : Inport  Port=4
  l : Inport  Port=5
  ml : Inport  Port=6
  M_BAL : Inport  Port=7
  BALANCEO : Inport  Port=8
  theta(t) : Inport  Port=9
  Discrete-Time Integrator{2..5} (4 alike) : DiscreteIntegrator  SampleTime=-1  ICPrevOutput=DiscIntNeverNeededParam  ICPrevScaledInput=DiscIntNeverNeededParam
  Gain10 : Gain  Gain=1/rtd
  Gain18 : Gain  Gain=rtd
  Gain2 : Gain  Gain=KIt
  Gain3 : Gain  Gain=KDh
  Gain4 : Gain  Gain=KPh
  Gain5 : Gain  Gain=KIh
  Gain6 : Gain  Gain=KPt
  Gain7 : Gain  Gain=KDt
  Gain9 : Gain  Gain=2/rhd
  Rate Limiter1 : RateLimiter  RisingSlewLimit=vx_max/rtd  FallingSlewLimit=-vx_max/rtd  SampleTimeMode=inherited
  Saturation : Saturate  UpperLimit=vx_max/rtd  LowerLimit=-vx_max/rtd
  Subsystem : Subsystem
  Sum1 : Sum  Inputs=|+-
  Sum2 : Sum  Inputs=+++
  Sum4 : Sum  Inputs=|+-
  Sum5 : Sum  Inputs=+++
  Sum8 : Sum  Inputs=|+-
  Ttm_ : Outport
  Thm_ : Outport  Port=2
  xt* : Outport  Port=3
  wires:
  M_BAL/1 -> Subsystem/3(In3)
  theta(t)/1 -> Subsystem/5(In5)
  BALANCEO/1 -> Subsystem/4(In4)
  Gain2/1 -> Sum5/1
  l/1 -> Subsystem/1(l)
  ml/1 -> Subsystem/2(ml)
  Sum1/1 -> Discrete-Time Integrator5/1, Gain3/1
  Gain18/1 -> xt*/1
  Saturation/1 -> Rate Limiter1/1
  Sum8/1 -> Saturation/1
  Gain10/1 -> Sum8/1
  vXref/1 -> Gain10/1
  Rate Limiter1/1 -> Sum4/1, Gain18/1
  Gain6/1 -> Sum5/2
  vYref/1 -> Gain9/1
  Discrete-Time Integrator4/1 -> Gain5/1
  Discrete-Time Integrator2/1 -> Gain2/1
  Gain3/1 -> Sum2/3
  Gain7/1 -> Sum5/3
  Gain5/1 -> Sum2/1
  Gain4/1 -> Sum2/2
  Gain9/1 -> Sum1/1
  Sum4/1 -> Discrete-Time Integrator3/1, Gain7/1
  Discrete-Time Integrator5/1 -> Discrete-Time Integrator4/1, Gain4/1
  Discrete-Time Integrator3/1 -> Discrete-Time Integrator2/1, Gain6/1
  whd/1 -> Sum1/2
  wtd/1 -> Sum4/2
  Sum5/1 -> Ttm_/1  "Ttm_"
  Sum2/1 -> Thm_/1  "Thm_"
  Subsystem/1(vX_Balanceo) -> Sum8/2

== system Planta_15_9_24/Planta/Cable izaje elástico amortiguado ==
  note: l_h
  Fhw : Inport
  l(t) : Inport  Port=2
  Yt0 : Inport  Port=3
  xh(t) : Inport  Port=4
  Constant9 : Constant  Value=0
  Relational Operator : RelationalOperator  OutDataTypeStr=boolean  RndMeth=Simplest
  Sum : Sum  Inputs=|+-
  Switch1 : Switch  Criteria=u2 > Threshold
  Fhw(t) : Outport
  wires:
  l(t)/1 -> Relational Operator/1
  Sum/1 -> Relational Operator/2
  Fhw/1 -> Switch1/1
  Yt0/1 -> Sum/1
  Constant9/1 -> Switch1/3
  Relational Operator/1 -> Switch1/2
  xh(t)/1 -> Sum/2
  Switch1/1 -> Fhw(t)/1

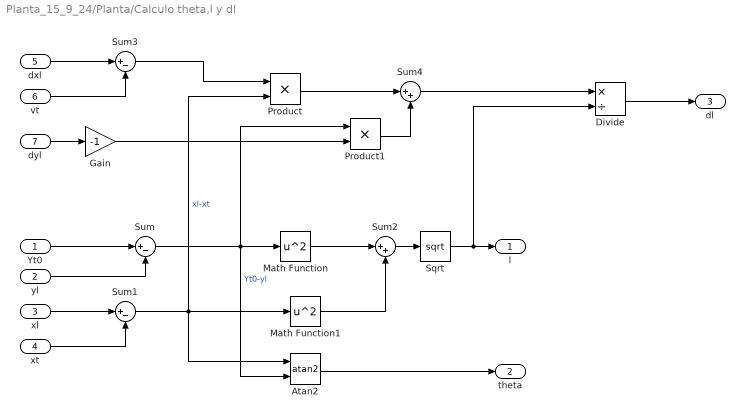
== system Planta_15_9_24/Planta/Calculo theta,l y dl ==
  Yt0 : Inport
  yl : Inport  Port=2
  xl : Inport  Port=3
  xt : Inport  Port=4
  dxl : Inport  Port=5
  vt : Inport  Port=6
  dyl : Inport  Port=7
  Atan2 : Trigonometry  Operator=atan2
  Divide : Product  Inputs=*/
  Gain : Gain  Gain=-1
  Math Function : Math  Operator=square  SaturateOnIntegerOverflow=on
  Math Function1 : Math  Operator=square  SaturateOnIntegerOverflow=on
  Product : Product
  Product1 : Product
  Sqrt : Sqrt  SaturateOnIntegerOverflow=on
  Sum : Sum  Inputs=|+-
  Sum1 : Sum  Inputs=|+-
  Sum2 : Sum  Inputs=|++
  Sum3 : Sum  Inputs=|+-
  Sum4 : Sum  Inputs=|++
  l : Outport
  theta : Outport  Port=2
  dl : Outport  Port=3
  wires:
  Yt0/1 -> Sum/1
  yl/1 -> Sum/2
  xl/1 -> Sum1/1
  xt/1 -> Sum1/2
  Atan2/1 -> theta/1
  Sum1/1 -> Product/2, Math Function1/1, Atan2/1  "xl-xt"
  Sum/1 -> Product1/1, Atan2/2, Math Function/1  "Yt0-yl"
  Math Function/1 -> Sum2/1
  Math Function1/1 -> Sum2/2
  Sum2/1 -> Sqrt/1
  Sqrt/1 -> Divide/2, l/1
  dxl/1 -> Sum3/1
  vt/1 -> Sum3/2
  Sum3/1 -> Product/1
  dyl/1 -> Gain/1
  Gain/1 -> Product1/2
  Product/1 -> Sum4/1
  Product1/1 -> Sum4/2
  Sum4/1 -> Divide/1
  Divide/1 -> dl/1

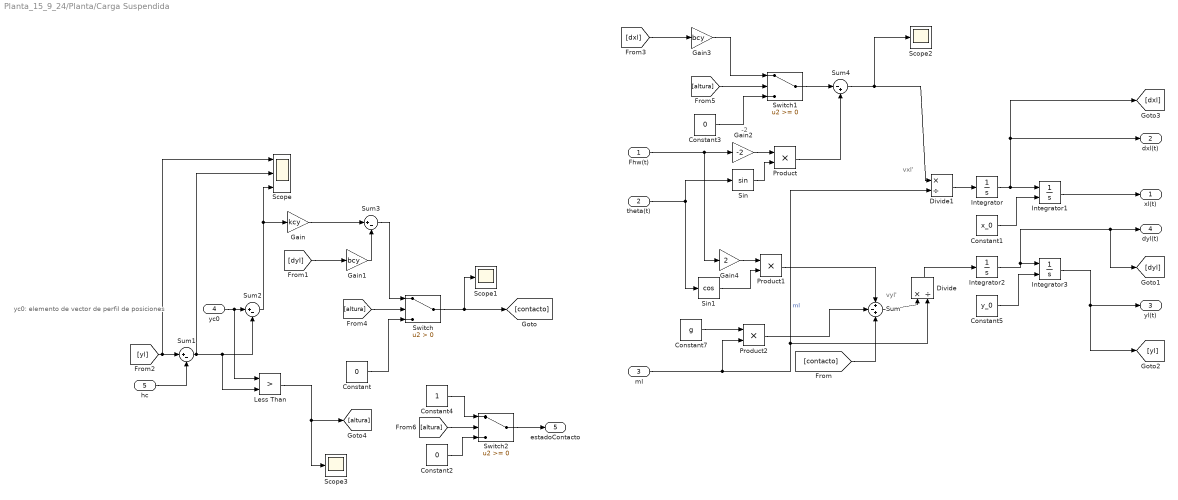
== system Planta_15_9_24/Planta/Carga Suspendida ==
  note: -2
  note: vxl'
  note: vyl'
  note: yc0: elemento de vector de perfil de posiciones
  Fhw(t) : Inport
  theta(t) : Inport  Port=2
  ml : Inport  Port=3
  yc0 : Inport  Port=4
  hc : Inport  Port=5
  Constant : Constant  Value=0
  Constant1 : Constant  Value=x_0
  Constant2 : Constant  Value=0
  Constant3 : Constant  Value=0
  Constant4 : Constant
  Constant5 : Constant  Value=y_0
  Constant7 : Constant  Value=g
  Divide : Product  Inputs=*/
  Divide1 : Product  Inputs=*/
  Gain : Gain  Gain=kcy
  Gain1 : Gain  Gain=bcy
  Gain2 : Gain  Gain=-2
  Gain3 : Gain  Gain=bcy
  Gain4 : Gain  Gain=2
  Integrator : Integrator
  Integrator1 : Integrator  InitialConditionSource=external
  Integrator2 : Integrator
  Integrator3 : Integrator  InitialConditionSource=external
  Less Than : RelationalOperator  Operator=>  OutDataTypeStr=boolean  RndMeth=Simplest
  Product : Product
  Product1 : Product
  Product2 : Product
  Scope : Scope  NumInputPorts=3
  Scope1 : Scope
  Scope2 : Scope
  Scope3 : Scope
  Sin : Trigonometry
  Sin1 : Trigonometry  Operator=cos
  Sum : Sum  Inputs=+-+
  Sum1 : Sum  Inputs=|+-
  Sum2 : Sum  Inputs=|+-
  Sum3 : Sum  Inputs=|+-
  Sum4 : Sum  Inputs=|-+
  Switch : Switch  Criteria=u2 > Threshold
  Switch1 : Switch
  Switch2 : Switch
  xl(t) : Outport
  dxl(t) : Outport  Port=2
  yl(t) : Outport  Port=3
  dyl(t) : Outport  Port=4
  estadoContacto : Outport  Port=5
  wires:
  Divide1/1 -> Integrator/1
  theta(t)/1 -> Sin1/1, Sin/1
  Constant7/1 -> Product2/1
  Product2/1 -> Sum/2
  Product/1 -> Sum4/2
  Fhw(t)/1 -> Gain4/1, Gain2/1
  Sum/1 -> Divide/1
  Integrator/1 -> [dxl], dxl(t)/1, Integrator1/1
  Sin1/1 -> Product1/2
  Gain2/1 -> Product/1
  Product1/1 -> Sum/1
  Sin/1 -> Product/2
  Integrator1/1 -> xl(t)/1
  Integrator2/1 -> [dyl], dyl(t)/1, Integrator3/1
  Divide/1 -> Integrator2/1
  Gain4/1 -> Product1/1
  Integrator3/1 -> [yl], yl(t)/1
  ml/1 -> Product2/2, Divide1/2, Divide/2  "ml"
  [yl] -> Scope/1, Sum1/1
  hc/1 -> Sum1/2
  Sum1/1 -> Scope/2, Less Than/2, Sum2/2
  yc0/1 -> Less Than/1, Sum2/1
  Constant/1 -> Switch/3
  [dyl] -> Gain1/1
  Gain1/1 -> Sum3/2
  Gain/1 -> Sum3/1
  Sum2/1 -> Scope/3, Gain/1
  Sum3/1 -> Switch/1
  Switch/1 -> Scope1/1, [contacto]
  [contacto] -> Sum/3
  Constant1/1 -> Integrator1/2
  [dxl] -> Gain3/1
  [altura] -> Switch/2
  [altura] -> Switch1/2
  Constant3/1 -> Switch1/3
  Gain3/1 -> Switch1/1
  Switch1/1 -> Sum4/1
  Sum4/1 -> Scope2/1, Divide1/1
  Switch2/1 -> estadoContacto/1
  Constant2/1 -> Switch2/3
  Constant4/1 -> Switch2/1
  [altura] -> Switch2/2
  Constant5/1 -> Integrator3/2
  Less Than/1 -> Scope3/1, [altura]

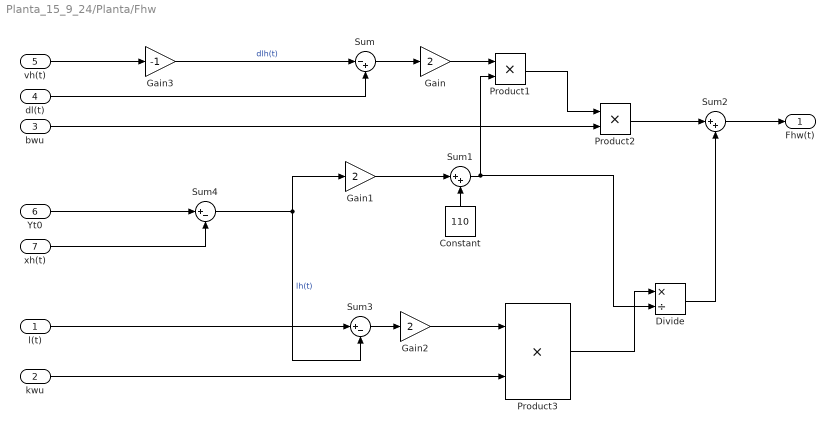
== system Planta_15_9_24/Planta/Fhw ==
  l(t) : Inport
  kwu : Inport  Port=2
  bwu : Inport  Port=3
  dl(t) : Inport  Port=4
  vh(t) : Inport  Port=5
  Yt0 : Inport  Port=6
  xh(t) : Inport  Port=7
  Constant : Constant  Value=110
  Divide : Product  Inputs=*/
  Gain : Gain  Gain=2
  Gain1 : Gain  Gain=2
  Gain2 : Gain  Gain=2
  Gain3 : Gain  Gain=-1
  Product1 : Product
  Product2 : Product
  Product3 : Product
  Sum : Sum  Inputs=|-+
  Sum1 : Sum  Inputs=|++
  Sum2 : Sum  Inputs=|++
  Sum3 : Sum  Inputs=|+-
  Sum4 : Sum  Inputs=|+-
  Fhw(t) : Outport
  wires:
  dl(t)/1 -> Sum/2
  Sum/1 -> Gain/1
  Gain1/1 -> Sum1/1
  Sum4/1 -> Sum3/2, Gain1/1  "lh(t)"
  l(t)/1 -> Sum3/1
  Constant/1 -> Sum1/2
  Gain/1 -> Product1/1
  Sum1/1 -> Product1/2, Divide/2
  Product1/1 -> Product2/1
  bwu/1 -> Product2/2
  Product2/1 -> Sum2/1
  Sum3/1 -> Gain2/1
  Gain2/1 -> Product3/1
  kwu/1 -> Product3/2
  Product3/1 -> Divide/1
  Divide/1 -> Sum2/2
  Sum2/1 -> Fhw(t)/1
  vh(t)/1 -> Gain3/1
  Gain3/1 -> Sum/1  "dlh(t)"
  Yt0/1 -> Sum4/1
  xh(t)/1 -> Sum4/2

== system Planta_15_9_24/Planta/Freno Izaje ==
  pulsadorBEh : Inport
  pulsadorBh : Inport  Port=2
  whm : Inport  Port=3
  whd : Inport  Port=4
  Constant3 : Constant  Value=0
  Constant6 : Constant  Value=0
  Gain1 : Gain  Gain=-bhEb
  Gain9 : Gain  Gain=-bhb
  Saturation : Saturate  UpperLimit=Thb_Max  LowerLimit=-Thb_Max
  Saturation1 : Saturate  UpperLimit=ThEb_Max  LowerLimit=-ThEb_Max
  Scope : Scope  NumInputPorts=2
  Switch : Switch  Criteria=u2 > Threshold
  Switch1 : Switch  Criteria=u2 > Threshold
  Thb : Outport  VectorParamsAs1DForOutWhenUnconnected=off
  ThEb : Outport  Port=2  VectorParamsAs1DForOutWhenUnconnected=off
  wires:
  Switch/1 -> Scope/1, Thb/1
  pulsadorBh/1 -> Switch/2
  pulsadorBEh/1 -> Switch1/2
  Switch1/1 -> Scope/2, ThEb/1
  Gain9/1 -> Saturation/1
  whm/1 -> Gain9/1
  Saturation/1 -> Switch/1
  Constant3/1 -> Switch/3
  Constant6/1 -> Switch1/3
  Saturation1/1 -> Switch1/1
  Gain1/1 -> Saturation1/1
  whd/1 -> Gain1/1

== system Planta_15_9_24/Planta/Freno carro ==
  wtm : Inport
  pulsadorTb : Inport  Port=2
  Constant3 : Constant  Value=0
  Gain9 : Gain  Gain=-btb
  Saturation : Saturate  UpperLimit=Ttb_Max  LowerLimit=-Ttb_Max
  Scope : Scope
  Switch : Switch  Criteria=u2 > Threshold
  Ttb : Outport  VectorParamsAs1DForOutWhenUnconnected=off
  wires:
  wtm/1 -> Gain9/1
  Saturation/1 -> Switch/1
  Switch/1 -> Scope/1, Ttb/1
  pulsadorTb/1 -> Switch/2
  Constant3/1 -> Switch/3
  Gain9/1 -> Saturation/1

== system Planta_15_9_24/Planta/Ftw ==
  xtd(t) : Inport
  xt(t) : Inport  Port=2
  vtd(t) : Inport  Port=3
  vt(t) : Inport  Port=4
  Gain1 : Gain  Gain=Ktw
  Gain2 : Gain  Gain=btw
  Sum : Sum
  Sum1 : Sum  Inputs=|+-
  Sum2 : Sum  Inputs=|+-
  Ftw(t) : Outport
  wires:
  Sum2/1 -> Gain2/1
  xtd(t)/1 -> Sum1/1
  vt(t)/1 -> Sum2/2
  xt(t)/1 -> Sum1/2
  Sum/1 -> Ftw(t)/1
  vtd(t)/1 -> Sum2/1
  Gain2/1 -> Sum/2
  Gain1/1 -> Sum/1
  Sum1/1 -> Gain1/1

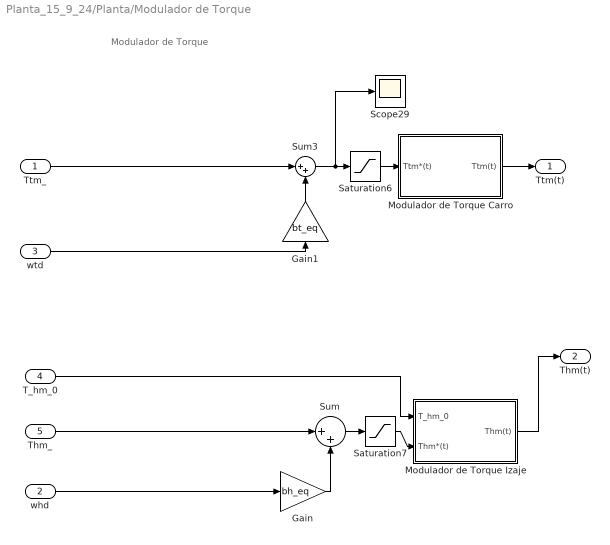
== system Planta_15_9_24/Planta/Modulador de Torque ==
  note: Modulador de Torque
  Ttm_ : Inport
  whd : Inport  Port=2
  wtd : Inport  Port=3
  T_hm_0 : Inport  Port=4
  Thm_ : Inport  Port=5
  Gain : Gain  Gain=bh_eq
  Gain1 : Gain  Gain=bt_eq
  Modulador de Torque Carro : Subsystem
  Modulador de Torque Izaje : Subsystem
  Saturation6 : Saturate  UpperLimit=Ttm_Max  LowerLimit=-Ttm_Max
  Saturation7 : Saturate  UpperLimit=Thm_Max  LowerLimit=-Thm_Max
  Scope29 : Scope
  Sum : Sum  Inputs=|++
  Sum3 : Sum  Inputs=|++
  Ttm(t) : Outport
  Thm(t) : Outport  Port=2
  wires:
  T_hm_0/1 -> Modulador de Torque Izaje/1(T_hm_0)
  Gain/1 -> Sum/2
  Sum/1 -> Saturation7/1
  wtd/1 -> Gain1/1
  Saturation6/1 -> Modulador de Torque Carro/1(Ttm*(t))
  Saturation7/1 -> Modulador de Torque Izaje/2(Thm*(t))
  Sum3/1 -> Scope29/1, Saturation6/1
  Gain1/1 -> Sum3/2
  Ttm_/1 -> Sum3/1
  Modulador de Torque Izaje/1(Thm(t)) -> Thm(t)/1
  whd/1 -> Gain/1
  Modulador de Torque Carro/1(Ttm(t)) -> Ttm(t)/1
  Thm_/1 -> Sum/1

== system Planta_15_9_24/Planta/Subsistema Carro ==
  theta(t) : Inport
  Fhw(t) : Inport  Port=2
  Ftw(t) : Inport  Port=3
  Constant : Constant  Value=x_0
  Gain : Gain  Gain=1/Mt
  Gain1 : Gain  Gain=2
  Gain2 : Gain  Gain=bt
  Integrator : Integrator
  Integrator1 : Integrator  InitialConditionSource=external
  Product : Product
  Sin : Trigonometry
  Sum : Sum  Inputs=++-
  xt(t) : Outport
  vt(t) : Outport  Port=2
  at(t) : Outport  Port=3
  wires:
  Integrator/1 -> vt(t)/1, Integrator1/1, Gain2/1
  Gain1/1 -> Product/2
  theta(t)/1 -> Sin/1
  Sum/1 -> Gain/1
  Product/1 -> Sum/1
  Integrator1/1 -> xt(t)/1
  Ftw(t)/1 -> Sum/2
  Gain2/1 -> Sum/3
  Fhw(t)/1 -> Gain1/1
  Sin/1 -> Product/1
  Constant/1 -> Integrator1/2
  Gain/1 -> at(t)/1, Integrator/1

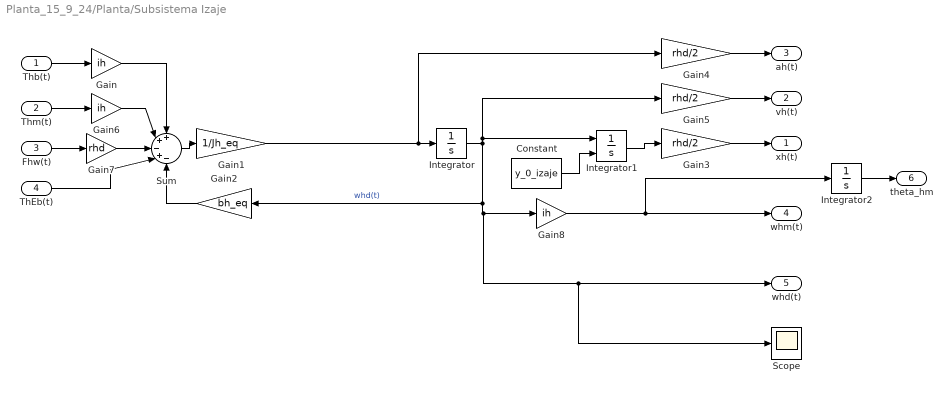
== system Planta_15_9_24/Planta/Subsistema Izaje ==
  Thb(t) : Inport
  Thm(t) : Inport  Port=2
  Fhw(t) : Inport  Port=3
  ThEb(t) : Inport  Port=4
  Constant : Constant  Value=y_0_izaje
  Gain : Gain  Gain=ih
  Gain1 : Gain  Gain=1/Jh_eq
  Gain2 : Gain  Gain=bh_eq
  Gain3 : Gain  Gain=rhd/2
  Gain4 : Gain  Gain=rhd/2
  Gain5 : Gain  Gain=rhd/2
  Gain6 : Gain  Gain=ih
  Gain7 : Gain  Gain=rhd
  Gain8 : Gain  Gain=ih
  Integrator : Integrator
  Integrator1 : Integrator  InitialConditionSource=external
  Integrator2 : Integrator
  Scope : Scope
  Sum : Sum  Inputs=++-+-
  xh(t) : Outport
  vh(t) : Outport  Port=2
  ah(t) : Outport  Port=3
  whm(t) : Outport  Port=4
  whd(t) : Outport  Port=5
  theta_hm : Outport  Port=6
  wires:
  Integrator/1 -> Gain5/1, Integrator1/1, Scope/1, whd(t)/1, Gain8/1, Gain2/1  "whd(t)"
  Gain2/1 -> Sum/5
  Gain4/1 -> ah(t)/1
  Gain3/1 -> xh(t)/1
  Gain5/1 -> vh(t)/1
  Fhw(t)/1 -> Gain7/1
  Integrator1/1 -> Gain3/1
  Thb(t)/1 -> Gain/1
  Sum/1 -> Gain1/1
  Thm(t)/1 -> Gain6/1
  Gain/1 -> Sum/1
  Gain6/1 -> Sum/2
  Gain7/1 -> Sum/3
  ThEb(t)/1 -> Sum/4
  Gain8/1 -> Integrator2/1, whm(t)/1
  Constant/1 -> Integrator1/2
  Gain1/1 -> Gain4/1, Integrator/1
  Integrator2/1 -> theta_hm/1
